simulink model "Pulse_Generator"  (R2022b)
settings: Solver=VariableStepAuto  StartTime=0.0  StopTime=0.002  RelTol=1e-3
libraries: spsOnDelayLib x2
settings Model: Creator=Hyeongmeen Baik  LastModifiedBy=Hyeongmeen Baik

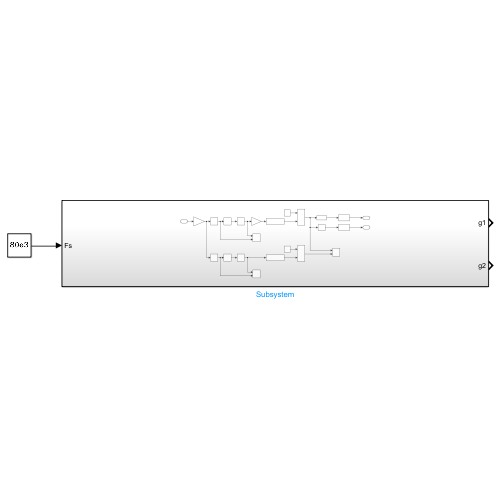
[thumbnail: Simulink's stored preview of the top-level diagram]
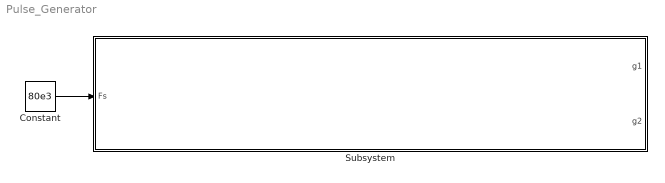
== system Pulse_Generator ==
  Constant : Constant  Value=80e3
  Subsystem : Subsystem
  wires:
  Constant/1 -> Subsystem/1(Fs)

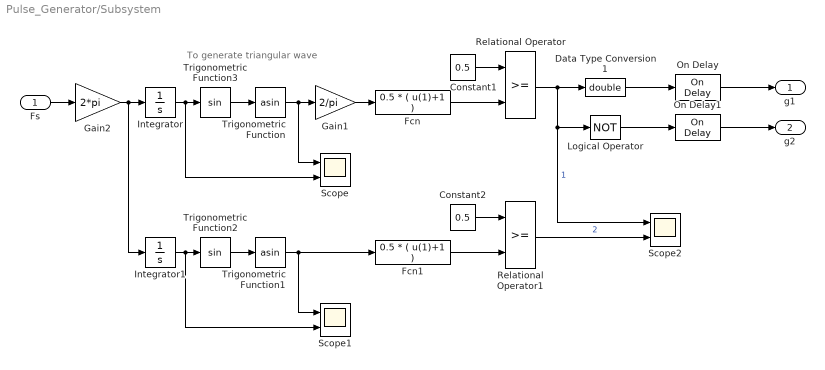
== system Pulse_Generator/Subsystem ==
  note: To generate triangular wave
  Fs : Inport
  Constant1 : Constant  Value=0.5
  Constant2 : Constant  Value=0.5
  Data Type Conversion1 : DataTypeConversion  OutDataTypeStr=double  SaturateOnIntegerOverflow=off  RndMeth=Floor
  Fcn : Fcn  Expr=0.5 * ( u(1)+1 )
  Fcn1 : Fcn  Expr=0.5 * ( u(1)+1 )
  Gain1 : Gain  Gain=2/pi  SaturateOnIntegerOverflow=on  OutDataTypeStr=Inherit: Same as input  ParamDataTypeStr=Inherit: Same as input
  Gain2 : Gain  Gain=2*pi  SaturateOnIntegerOverflow=on  OutDataTypeStr=Inherit: Same as input  ParamDataTypeStr=Inherit: Same as input
  Integrator : Integrator
  Integrator1 : Integrator
  Logical Operator : Logic  Operator=NOT  AllPortsSameDT=off  OutDataTypeStr=float('double')
  On Delay : spsOnDelayLib/On Delay  DelayType=On delay  delay=400e-9  ic=0  Ts=0
  On Delay1 : spsOnDelayLib/On Delay  DelayType=On delay  delay=400e-9  ic=0  Ts=0
  Relational Operator : RelationalOperator  OutDataTypeStr=boolean  InputSameDT=off
  Relational Operator1 : RelationalOperator  OutDataTypeStr=boolean  InputSameDT=off
  Scope : Scope  NumInputPorts=2
  Scope1 : Scope  NumInputPorts=2
  Scope2 : Scope  NumInputPorts=2
  Trigonometric Function : Trigonometry  Operator=asin
  Trigonometric Function1 : Trigonometry  Operator=asin
  Trigonometric Function2 : Trigonometry
  Trigonometric Function3 : Trigonometry
  g1 : Outport
  g2 : Outport  Port=2
  wires:
  Fs/1 -> Gain2/1
  Integrator/1 -> Scope/2, Trigonometric Function3/1
  On Delay1/1 -> g2/1
  Trigonometric Function3/1 -> Trigonometric Function/1
  Fcn/1 -> Relational Operator/2
  Logical Operator/1 -> On Delay1/1
  Gain1/1 -> Fcn/1
  Data Type Conversion1/1 -> On Delay/1
  Trigonometric Function/1 -> Scope/1, Gain1/1
  On Delay/1 -> g1/1
  Constant1/1 -> Relational Operator/1
  Relational Operator/1 -> Data Type Conversion1/1, Scope2/1, Logical Operator/1  "1"
  Integrator1/1 -> Scope1/2, Trigonometric Function2/1
  Gain2/1 -> Integrator1/1, Integrator/1
  Trigonometric Function1/1 -> Fcn1/1, Scope1/1
  Trigonometric Function2/1 -> Trigonometric Function1/1
  Fcn1/1 -> Relational Operator1/2
  Constant2/1 -> Relational Operator1/1
  Relational Operator1/1 -> Scope2/2  "2"
